simulink model "TV2016_CAN"  (Simulink 8.5)
settings: Solver=ode1  StartTime=0.0  StopTime=inf  FixedStep=0.001  RelTol=1e-3
PreLoadFcn:
  | FSE_Parameters
values from neighbouring files (symbols this model uses):
  car_params = Simulink_Car_params    [TV2016_parameters.m]
  i_Diff = 15.47    [TV2016_parameters.m]
  Kp = 1    [TV2016_parameters.m]
  settings = Simulink_Settings    [TV2016_parameters.m]
  SpdC_BCC = 0    [TV2016_parameters.m]
  Speed_Neg_sat = -21    [TV2016_parameters.m]
  Speed_Pos_sat = 21    [TV2016_parameters.m]
  Tn_n = 0    [TV2016_parameters.m]
  Use_Joystick = 1    [TV2016_parameters.m]
undefined symbols (not defined in the file or in its folder): canChannel
libraries: CarMaker4SL x139, simulink x18, canmsglib x10, simulink_extras x7, canlib x5, sldrtlib x1
(part 4 of 4)

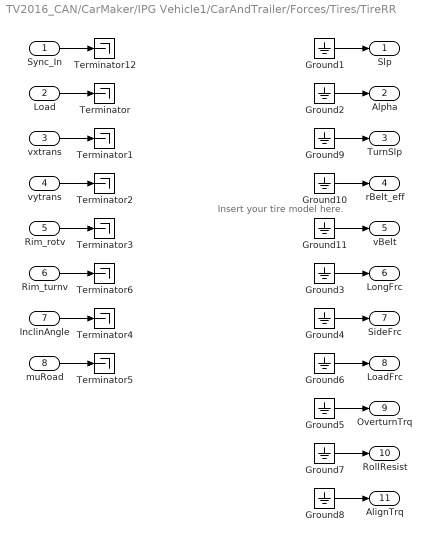
== system TV2016_CAN/CarMaker/IPG Vehicle1/CarAndTrailer/Forces/Tires/TireRR ==
  note: Insert your tire model here.
  Sync_In : Inport
  Load : Inport  Port=2
  vxtrans : Inport  Port=3
  vytrans : Inport  Port=4
  Rim_rotv : Inport  Port=5
  Rim_turnv : Inport  Port=6
  InclinAngle : Inport  Port=7
  muRoad : Inport  Port=8
  Ground{1..11} (11 alike) : Ground
  Terminator{,1..6,12} (8 alike) : Terminator
  Slp : Outport
  Alpha : Outport  Port=2
  TurnSlp : Outport  Port=3
  rBelt_eff : Outport  Port=4
  vBelt : Outport  Port=5
  LongFrc : Outport  Port=6
  SideFrc : Outport  Port=7
  LoadFrc : Outport  Port=8
  OverturnTrq : Outport  Port=9
  RollResist : Outport  Port=10
  AlignTrq : Outport  Port=11
  wires:
  Ground11/1 -> vBelt/1
  Ground10/1 -> rBelt_eff/1
  Ground9/1 -> TurnSlp/1
  Rim_turnv/1 -> Terminator6/1
  Sync_In/1 -> Terminator12/1
  Ground2/1 -> Alpha/1
  Ground3/1 -> LongFrc/1
  Ground4/1 -> SideFrc/1
  Ground5/1 -> OverturnTrq/1
  vxtrans/1 -> Terminator1/1
  vytrans/1 -> Terminator2/1
  Rim_rotv/1 -> Terminator3/1
  InclinAngle/1 -> Terminator4/1
  muRoad/1 -> Terminator5/1
  Load/1 -> Terminator/1
  Ground1/1 -> Slp/1
  Ground6/1 -> LoadFrc/1
  Ground7/1 -> RollResist/1
  Ground8/1 -> AlignTrq/1

== matlab function CarMaker/VehicleControl1/CreateBus VhclCtrl/Add KERS ==
  data: brake_pedal input double; KERS_pos output double; brake_pos output double
function [KERS_pos, brake_pos] = fcn(brake_pedal)
%#codegen

% 0-0.5 = KERS , 0.5-1.0 = 0-1 brake
    KERS_pos = single(0);
    brake_pos = 0;
    if brake_pedal >= 0 & brake_pedal <=  0.5
        KERS_pos = single(2*brake_pedal);
        brake_pos = 0;
    else
        KERS_pos = single(1);
        brake_pos = 2*(brake_pedal -0.5);
    end
    
%     if brake_pedal >= 0 & brake_pedal <=  1.0001
%         KERS_pos = single(brake_pedal);
%         brake_pos = 0;
%     else
%         KERS_pos = single(1);
%         brake_pos = 2*(brake_pedal -0.5);
%     end


end

== matlab function CarMaker/Function-Call Subsystem4/MATLAB Function1 ==
  data: trq_pos_16 input double; trq_pos_f output double; trq_neg_16 input double; w_set_16 input double; trq_neg_f output double; w_set_f output double; settings parameter double
function [trq_pos_f, trq_neg_f, w_set_f] = fcn(trq_pos_16, trq_neg_16, w_set_16, settings)
%#codegen

Sf = 0.0098;
trq_pos_f = double( trq_pos_16*Sf);
trq_neg_f = double( trq_neg_16*Sf);
w_set_f = double( w_set_16);

== matlab function CarMaker/Function-Call Subsystem4/MATLAB Function2 ==
  data: trq_pos_16 input double; trq_pos_f output double; trq_neg_16 input double; w_set_16 input double; trq_neg_f output double; w_set_f output double; settings parameter double
function [trq_pos_f, trq_neg_f, w_set_f] = fcn(trq_pos_16, trq_neg_16, w_set_16, settings)
%#codegen

Sf = 0.0098;
trq_pos_f = double( trq_pos_16*Sf);
trq_neg_f = double( trq_neg_16*Sf);
w_set_f = double( w_set_16);

== matlab function CarMaker/Function-Call Subsystem4/MATLAB Function3 ==
  data: trq_pos_16 input double; trq_pos_f output double; trq_neg_16 input double; w_set_16 input double; trq_neg_f output double; w_set_f output double; settings parameter double
function [trq_pos_f, trq_neg_f, w_set_f] = fcn(trq_pos_16, trq_neg_16, w_set_16, settings)
%#codegen

Sf = 0.0098;
trq_pos_f = double( trq_pos_16*Sf);
trq_neg_f = double( trq_neg_16*Sf);
w_set_f = double( w_set_16);

== matlab function CarMaker/Sensors 1/"Measured Power"/MATLAB Function ==
  data: RPM_FL_IN input double; RPM_FR_IN input double; RPM_RL_IN input double; RPM_RR_IN input double; Pm_FL output double; T input double; T_FL output double; RPM_FL output double; Pm_FR output double; T_FR output double; RPM_FR output double; Pm_RL output double; T_RL output double; RPM_RL output double; Pm_RR output double; T_RR output double; RPM_RR output double
function [Pm_FL, T_FL, RPM_FL,Pm_FR, T_FR, RPM_FR,Pm_RL, T_RL,...
          RPM_RL,Pm_RR, T_RR, RPM_RR] = powerMeasurement(RPM_FL_IN, RPM_FR_IN,RPM_RL_IN,RPM_RR_IN, T)
%#codegen

%Conversion from RPM to rad/s
c = single(2*pi/60);

T_FL = T.FL;
T_FR = T.FR;
T_RL = T.RL;
T_RR = T.RR;
RPM_FL = RPM_FL_IN;
RPM_FR = RPM_FR_IN;
RPM_RL = RPM_RL_IN;
RPM_RR = RPM_RR_IN;


Pm_FL = RPM_FL*c*T.FL;
Pm_FR = RPM_FR*c*T.FR;
Pm_RL = RPM_RL*c*T.RL;
Pm_RR = RPM_RR*c*T.RR;

== matlab function CarMaker/Function-Call Subsystem4/MATLAB Function ==
  data: trq_pos_16 input double; trq_pos_f output double; trq_neg_16 input double; w_set_16 input double; trq_neg_f output double; w_set_f output double; settings parameter double
function [trq_pos_f, trq_neg_f, w_set_f] = fcn(trq_pos_16, trq_neg_16, w_set_16, settings)
%#codegen

Sf = 0.0098;
trq_pos_f = double( trq_pos_16*Sf);
trq_neg_f = double( trq_neg_16*Sf);
w_set_f = double( w_set_16);

== matlab function CarMaker/VehicleControl1/CreateBus VhclCtrl/RacingwheelInterface/Add KERS ==
  data: brake_pedal input double; KERS_pos output double; brake_pos output double
function [KERS_pos, brake_pos] = fcn(brake_pedal)
%#codegen

% 0-0.5 = KERS , 0.5-1.0 = 0-1 brake
    KERS_pos = single(0);
    brake_pos = 0;
    if (brake_pedal > 0) && (brake_pedal <  0.5)
        KERS_pos = single(2*brake_pedal);
        brake_pos = 0;
    else
        KERS_pos = single(1);
        brake_pos = 2*(brake_pedal -0.5);
    end
    
%     if brake_pedal >= 0 & brake_pedal <=  1.0001
%         KERS_pos = single(brake_pedal);
%         brake_pos = 0;
%     else
%         KERS_pos = single(1);
%         brake_pos = 2*(brake_pedal -0.5);
%     end


end
